simulink model "Part01"  (R2023b)
settings: Solver=VariableStepAuto  StartTime=0.0  StopTime=10.0  RelTol=1e-3
settings Model: Creator=UseR  LastModifiedBy=UseR

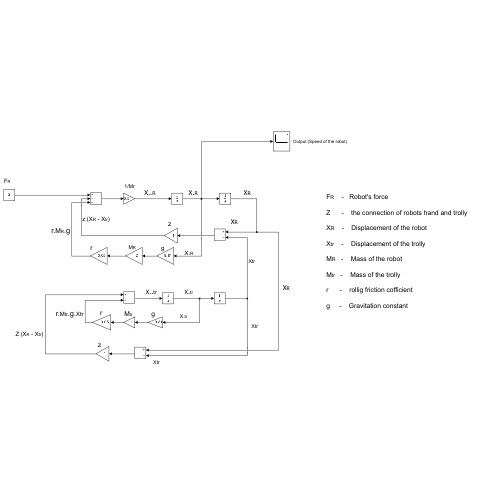
[thumbnail: Simulink's stored preview of the top-level diagram]
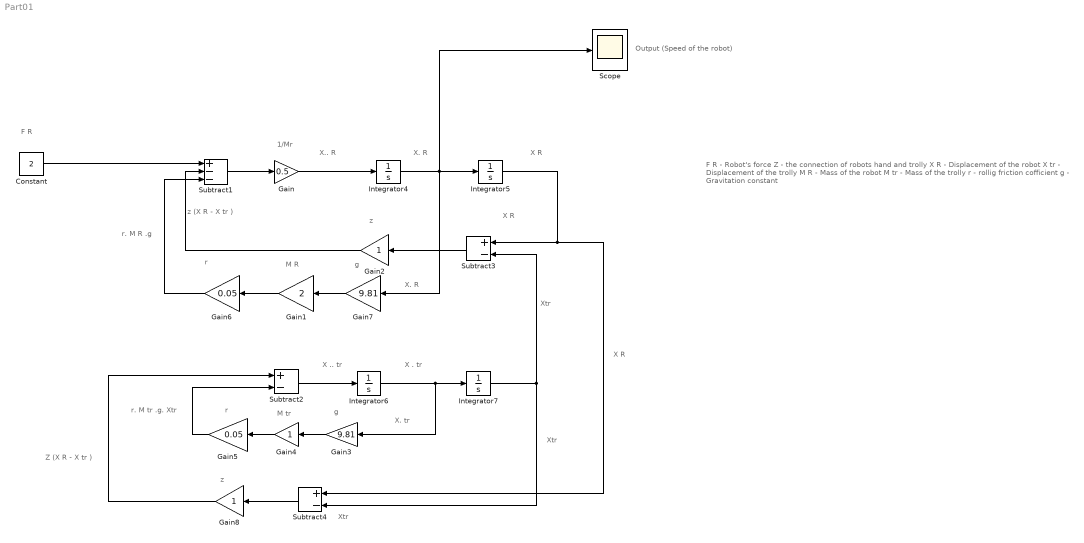
== system Part01 ==
  note: g
  note: r
  note: F R
  note: M tr
  note: r. M R .g
  note: Xtr
  note: Output (Speed of the robot)
  note: M R
  note: z
  note: z (X R - X tr )
  note: 1/Mr
  note: X.. R
  note: F R - Robot's force
      |
      | Z - the connection of robots hand and trolly
      |
      | X R - Displacement of the robot
      |
      | X tr - Displacement of the trolly
      |
      | M R - Mass of the robot
      |
      | M tr - Mass of the trolly
      |
      | r - rollig friction cofficient
      |
      | g - Gravitation constant
  note: Xtr
  note: X R
  note: Xtr
  note: X. R
  note: X R
  note: X . tr
  note: X R
  note: X. tr
  note: X. R
  note: r. M tr .g. Xtr
  note: g
  note: X .. tr
  note: Z (X R - X tr )
  note: r
  note: z
  Constant : Constant  Value=2
  Gain : Gain  Gain=0.5
  Gain1 : Gain  Gain=2
  Gain2 : Gain
  Gain3 : Gain  Gain=9.81
  Gain4 : Gain
  Gain5 : Gain  Gain=0.05
  Gain6 : Gain  Gain=0.05
  Gain7 : Gain  Gain=9.81
  Gain8 : Gain
  Integrator{4..7} (4 alike) : Integrator
  Scope : Scope
  Subtract1 : Sum  Inputs=+--
  Subtract2 : Sum  Inputs=+-
  Subtract3 : Sum  Inputs=+-
  Subtract4 : Sum  Inputs=+-
  wires:
  Integrator7/1 -> Subtract3/2, Subtract4/2
  Integrator4/1 -> Scope/1, Integrator5/1, Gain7/1
  Integrator5/1 -> Subtract3/1, Subtract4/1
  Gain5/1 -> Subtract2/2
  Gain3/1 -> Gain4/1
  Subtract3/1 -> Gain2/1
  Gain4/1 -> Gain5/1
  Integrator6/1 -> Integrator7/1, Gain3/1
  Gain7/1 -> Gain1/1
  Constant/1 -> Subtract1/1
  Subtract2/1 -> Integrator6/1
  Subtract4/1 -> Gain8/1
  Gain1/1 -> Gain6/1
  Gain8/1 -> Subtract2/1
  Subtract1/1 -> Gain/1
  Gain/1 -> Integrator4/1
  Gain2/1 -> Subtract1/2
  Gain6/1 -> Subtract1/3
